simulink model "SolarPowerComp"  (R2024b)
settings: Solver=VariableStepAuto  StartTime=0.0  StopTime=10  RelTol=1e-3
undefined symbols (not defined in the file): Acid, Lead
libraries: spsSeriesRLCBranchLib x8, spsCurrentMeasurementLib x3, spsPWMGeneratorDCDCLib x2, spsDiodeLib x2, spsMosfetLib x2, spsVoltageMeasurementLib x2, spsBatteryLib x1, spsGroundLib x1, spsPVArrayLib x1, sps_lib x1
settings Model: Creator=joshbenner  LastModifiedBy=joshbenner
settings SolverCC: ZeroCrossAlgorithm=Adaptive
settings DebuggingCC: MaskedZcDiagnostic=none  IgnoredZcDiagnostic=none

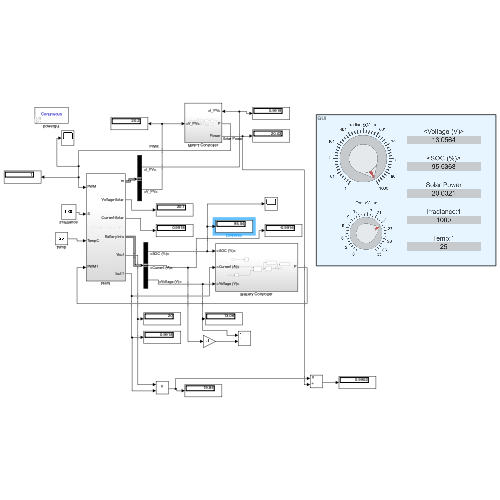
[thumbnail: Simulink's stored preview of the top-level diagram]
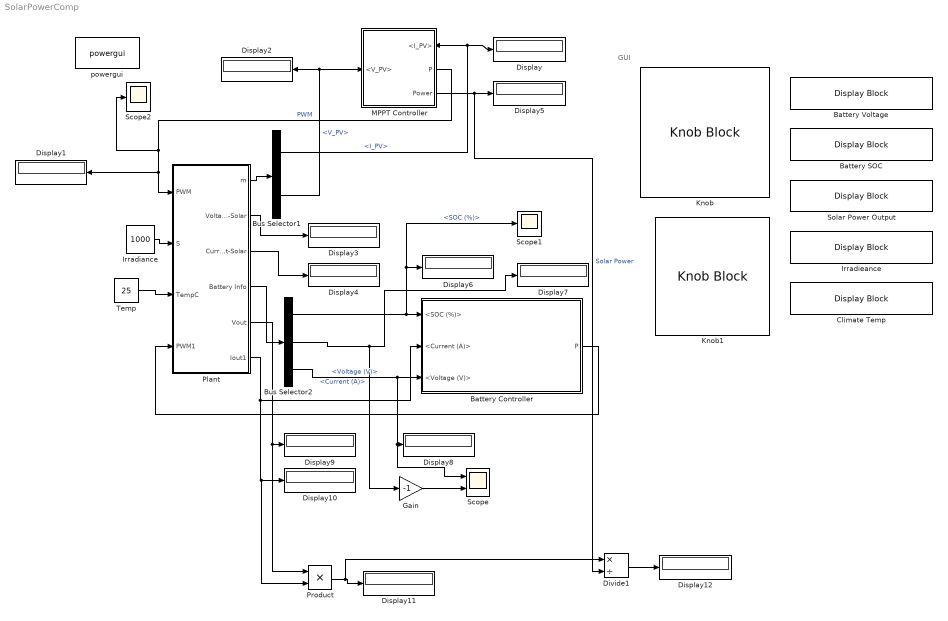
== system SolarPowerComp ==
  note: GUI
  Battery Controller : Subsystem
  Battery SOC : DisplayBlock  Transparency=1
  Battery Voltage : DisplayBlock  Transparency=1
  Bus Selector1 : BusSelector  OutputSignals=I_PV,V_PV
  Bus Selector2 : BusSelector  OutputSignals=SOC (%),Current (A),Voltage (V)
  Climate Temp : DisplayBlock  Transparency=1
  Display{,1..12} (13 alike) : Display
  Divide1 : Product  Inputs=*/
  Gain : Gain  Gain=-1
  Irradiance : Constant  Value=1000
  Irradieance : DisplayBlock  Transparency=1
  Knob : KnobBlock  ScaleMin=1  ScaleMax=1000
  Knob1 : KnobBlock  ScaleMax=35
  MPPT Controller : Subsystem
      settings: PortSchema="{\"entries\":[{\"content\":{\"sides\":[{\"content\":{\"connectorIds\":[\"In1\"]},\"type\":\"ConnectorPlacement.EquallySpacedRectSide\",\"uuid\":\"d3d26d18-f1d7-4526-bab1-51f87aba0634\"},{\"content\":{\"connectorIds\":[\"In2\",\"Out1\",\"Out2\"],\"side\":\"RIGHT\"},\"type\":\"ConnectorPlacement.EquallySpacedRectSide\",\"uuid\":\"345d964f-69df-4ff4-99f4-8db1e101ec0e\"},{\"content\":{\"side\":\"TOP\"},\"type\":\"ConnectorPlacement.EquallySpacedRectSide\",\"uuid\":\"81ceea76-a4b6-4476-a125-099e7862c238\"}]},\"type\":\"ConnectorPlacement.EquallySpacedConnector\",\"uuid\":\"a527d310-72d2-41d9-baeb-0576d2e35a0d\"}],\"packageUris\":[\"http://schema.mathworks.com/mf0/Connector/R2020b\"],\"version\":\"1.0\"}"
  Plant : Subsystem
  Product : Product
  Scope : Scope  NumInputPorts=2
  Scope1 : Scope
  Scope2 : Scope
  Solar Power Output : DisplayBlock  Transparency=1
  Temp : Constant  Value=25
  powergui : sps_lib/powergui  Priority=1  SimulationMode=Continuous  SampleTime=1e-6  frequency=60  Iterations=50  frequencyindice=0  Pbase=100e6  ErrMax=1e-4  UnitsV=kV  UnitsW=MW  buscounter=0  FunctionMessages=off  echomessages=off  EnableUseOfTLC=off  CurrentSourceSwitches=off  DisableSnubberDevices=off  DisableRonSwitches=off  DisableVfSwitches=off  DisplayEquations=off  AutomaticDiscreteSolvers=off  SolverType=Tustin/Backward Euler (TBE)  Interpol=off  ExternalGateDelay=off  methode=off  Ts=100  x0status=blocks  SPID=on  SwTol=0  HookPort=off  NonlinearTolerance=1e-4  nMaxIteration=100  ContinueOnMaxIteration=off  RestoreLinks=warning  ResistiveCurrentMeasurement=off  Frange=[0:2:500]  Ylog=off  Xlog=on  ShowGrid=off  save=off  variable=ZData  structure=0  ZoomFFT=off  StartTime=0.0  cycles=1  DisplayStyle=1  fundamental=60  FreqAxis=off  MaxFrequency=1000  frequencyindicesteady=1  RmsSteady=1  display=off
  wires:
  Bus Selector1/2 -> MPPT Controller/1(<V_PV>), Display2/1  "<V_PV>"
  Bus Selector1/1 -> MPPT Controller/2(<I_PV>), Display/1  "<I_PV>"
  MPPT Controller/1(P) -> Scope2/1, Display1/1, Plant/1(PWM)  "PWM"
  Temp/1 -> Plant/3(TempC)
  Plant/1(m) -> Bus Selector1/1
  Irradiance/1 -> Plant/2(S)
  MPPT Controller/2(Power) -> Divide1/2, Display5/1  "Solar Power"
  Plant/2(Voltage-Solar) -> Display3/1
  Plant/3(Current-Solar) -> Display4/1
  Plant/4(Battery Info) -> Bus Selector2/1
  Bus Selector2/1 -> Battery Controller/1(<SOC (%)>), Scope1/1, Display6/1  "<SOC (%)>"
  Bus Selector2/2 -> Gain/1, Display7/1  "<Current (A)>"
  Bus Selector2/3 -> Battery Controller/3(<Voltage (V)>), Scope/1, Display8/1  "<Voltage (V)>"
  Battery Controller/1(P) -> Plant/4(PWM1)
  Plant/5(Vout) -> Product/1, Display9/1
  Plant/6(Iout1) -> Battery Controller/2(<Current (A)>), Product/2, Display10/1
  Gain/1 -> Scope/2
  Product/1 -> Divide1/1, Display11/1
  Divide1/1 -> Display12/1

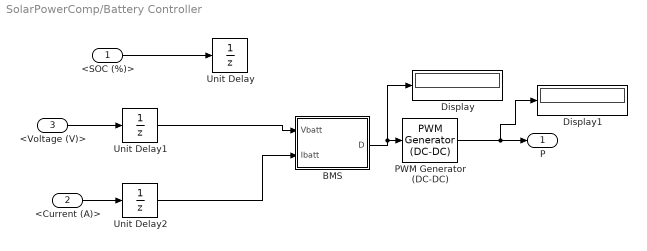
== system SolarPowerComp/Battery Controller ==
  <SOC (%)> : Inport
  <Current (A)> : Inport  Port=2
  <Voltage (V)> : Inport  Port=3
  BMS : MATLAB Function  TreatAsAtomicUnit=on
  Display : Display
  Display1 : Display
  PWM Generator (DC-DC) : spsPWMGeneratorDCDCLib/PWM Generator (DC-DC)  Fsw=100000  Ts=.000005
  Unit Delay : UnitDelay  SampleTime=-1  HasFrameUpgradeWarning=on
  Unit Delay1 : UnitDelay  SampleTime=-1  HasFrameUpgradeWarning=on
  Unit Delay2 : UnitDelay  SampleTime=-1  HasFrameUpgradeWarning=on
  P : Outport
  wires:
  PWM Generator (DC-DC)/1 -> Display1/1, P/1
  BMS/1(D) -> Display/1, PWM Generator (DC-DC)/1
  <SOC (%)>/1 -> Unit Delay/1
  <Voltage (V)>/1 -> Unit Delay1/1
  <Current (A)>/1 -> Unit Delay2/1
  Unit Delay1/1 -> BMS/1(Vbatt)
  Unit Delay2/1 -> BMS/2(Ibatt)

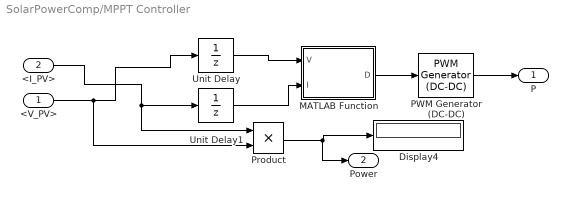
== system SolarPowerComp/MPPT Controller ==
  <V_PV> : Inport
  <I_PV> : Inport  Port=2
  Display4 : Display
  MATLAB Function : MATLAB Function  TreatAsAtomicUnit=on
  PWM Generator (DC-DC) : spsPWMGeneratorDCDCLib/PWM Generator (DC-DC)  Fsw=100000  Ts=.000005
  Product : Product
  Unit Delay : UnitDelay  SampleTime=-1  HasFrameUpgradeWarning=on
  Unit Delay1 : UnitDelay  SampleTime=-1  HasFrameUpgradeWarning=on
  P : Outport
  Power : Outport  Port=2
  wires:
  <V_PV>/1 -> Product/2, Unit Delay/1
  PWM Generator (DC-DC)/1 -> P/1
  <I_PV>/1 -> Product/1, Unit Delay1/1
  Unit Delay/1 -> MATLAB Function/1(V)
  MATLAB Function/1(D) -> PWM Generator (DC-DC)/1
  Product/1 -> Power/1, Display4/1
  Unit Delay1/1 -> MATLAB Function/2(I)

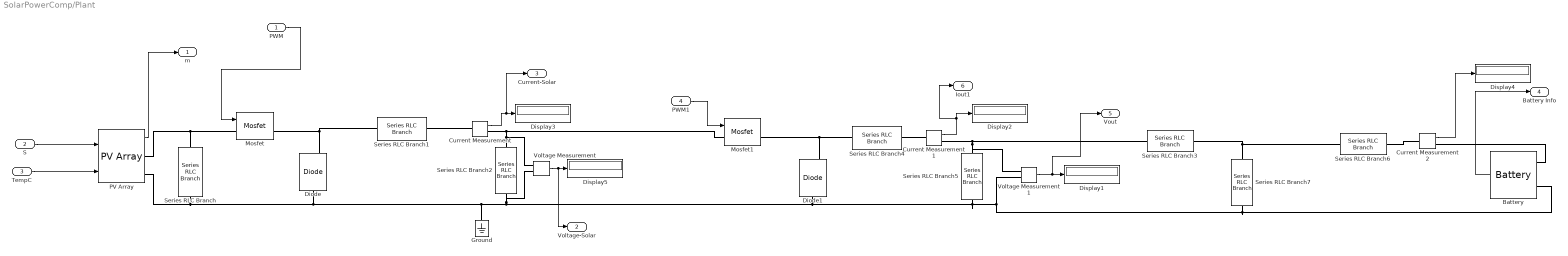
== system SolarPowerComp/Plant ==
  PWM : Inport
  S : Inport  Port=2
  TempC : Inport  Port=3
  PWM1 : Inport  Port=4
  Battery : spsBatteryLib/Battery  BatType=Lead-Acid  NomV=12  NomQ=5  SOC=95  Batt_Tr=1e-3  PresetModel=on  MaxQ=5.2083  MinV=9  FullV=13.0658  Dis_rate=1  R=0.024  Normal_OP=1.5514  expZone="[12.2171    0.0166667]"
  Current Measurement : spsCurrentMeasurementLib/Current Measurement  PhasorSimulation=off  OutputType=Complex  PSBequivalent=0
  Current Measurement1 : spsCurrentMeasurementLib/Current Measurement  PhasorSimulation=off  OutputType=Complex  PSBequivalent=0
  Current Measurement2 : spsCurrentMeasurementLib/Current Measurement  PhasorSimulation=off  OutputType=Complex  PSBequivalent=0
  Diode : spsDiodeLib/Diode  Ron=0.001  Lon=0  Vf=0.8  IC=0  UseSnubber=0  Rs=500  Cs=250e-9  Measurements=on
  Diode1 : spsDiodeLib/Diode  Ron=0.001  Lon=0  Vf=0.8  IC=0  UseSnubber=0  Rs=500  Cs=250e-9  Measurements=on
  Display{1..5} (5 alike) : Display
  Ground : spsGroundLib/Ground  LConnTagsString=a
  Mosfet : spsMosfetLib/Mosfet  Ron=0.1  Lon=0  Rd=0.01  Vfd=0  IC=0  Rs=1e5  Cs=inf  Measurements=on
  Mosfet1 : spsMosfetLib/Mosfet  Ron=0.1  Lon=0  Rd=0.01  Vfd=0  IC=0  Rs=1e5  Cs=inf  Measurements=on
  PV Array : spsPVArrayLib/PV Array  Npar=1  Nser=1  PlotType=one module @ 25 deg.C & specified irradiances  S_vec="[ 1000  500  100 ]"  Temp_C_vec="[ 45 25  ]"  ModuleName=User-defined  PlotWhenSelected=off  Pm=25.2  Ncell=60  Voc=22.41  Isc=1.54  Vm=18  Im=1.4  beta_Voc_pc=-0.36099  alpha_Isc_pc=0.102  beta_Voc=-0.080898  alpha_Isc=0.0015708  IL=1.5698  I0=5.9204e-11  nI=0.60755  Rsh=206.1422  Rs=1.1696  RobustModel=off  RobustCellTemperature=313.3991  BAL=on  Tc=1e-6  Tfilter=5e-5
  Series RLC Branch : spsSeriesRLCBranchLib/Series RLC Branch  LConnTagsString=__new0  RConnTagsString=__new0  BranchType=C  Resistance=.0001  Inductance=1e-3  SetiL0=off  InitialCurrent=0  Capacitance=1000e-6  Setx0=off  InitialVoltage=0  Measurements=None
  Series RLC Branch1 : spsSeriesRLCBranchLib/Series RLC Branch  LConnTagsString=__new0  RConnTagsString=__new0  BranchType=L  Resistance=.0001  Inductance=1e-3  SetiL0=off  InitialCurrent=0  Capacitance=1000e-6  Setx0=off  InitialVoltage=0  Measurements=None
  Series RLC Branch2 : spsSeriesRLCBranchLib/Series RLC Branch  LConnTagsString=__new0  RConnTagsString=__new0  BranchType=C  Resistance=.0001  Inductance=1e-3  SetiL0=off  InitialCurrent=0  Capacitance=20e-6  Setx0=off  InitialVoltage=0  Measurements=None
  Series RLC Branch3 : spsSeriesRLCBranchLib/Series RLC Branch  LConnTagsString=__new0  RConnTagsString=__new0  BranchType=R  Resistance=7  Inductance=1e-3  SetiL0=off  InitialCurrent=0  Capacitance=20e-6  Setx0=off  InitialVoltage=0  Measurements=None
  Series RLC Branch4 : spsSeriesRLCBranchLib/Series RLC Branch  LConnTagsString=__new0  RConnTagsString=__new0  BranchType=L  Resistance=.0001  Inductance=1e-3  SetiL0=off  InitialCurrent=0  Capacitance=1000e-6  Setx0=off  InitialVoltage=0  Measurements=None
  Series RLC Branch5 : spsSeriesRLCBranchLib/Series RLC Branch  LConnTagsString=__new0  RConnTagsString=__new0  BranchType=C  Resistance=.0001  Inductance=1e-3  SetiL0=off  InitialCurrent=0  Capacitance=20e-3  Setx0=off  InitialVoltage=0  Measurements=None
  Series RLC Branch6 : spsSeriesRLCBranchLib/Series RLC Branch  LConnTagsString=__new0  RConnTagsString=__new0  BranchType=R  Resistance=.0001  Inductance=1e-3  SetiL0=off  InitialCurrent=0  Capacitance=20e-6  Setx0=off  InitialVoltage=0  Measurements=None
  Series RLC Branch7 : spsSeriesRLCBranchLib/Series RLC Branch  LConnTagsString=__new0  RConnTagsString=__new0  BranchType=C  Resistance=.0001  Inductance=1e-3  SetiL0=off  InitialCurrent=0  Capacitance=4500e-6  Setx0=off  InitialVoltage=0  Measurements=None
  Voltage Measurement : spsVoltageMeasurementLib/Voltage Measurement  PhasorSimulation=off  OutputType=Complex  PSBequivalent=0
  Voltage Measurement1 : spsVoltageMeasurementLib/Voltage Measurement  PhasorSimulation=off  OutputType=Complex  PSBequivalent=0
  m : Outport
  Voltage-Solar : Outport  Port=2
  Current-Solar : Outport  Port=3
  Battery Info : Outport  Port=4
  Vout : Outport  Port=5
  Iout1 : Outport  Port=6
  wires:
  S/1 -> PV Array/1
  PV Array/1 -> m/1
  Voltage Measurement/1 -> Voltage-Solar/1, Display5/1
  TempC/1 -> PV Array/2
  PWM/1 -> Mosfet/1
  Current Measurement/1 -> Current-Solar/1, Display3/1
  PWM1/1 -> Mosfet1/1
  Voltage Measurement1/1 -> Vout/1, Display1/1
  Battery/1 -> Battery Info/1
  Current Measurement2/1 -> Display4/1
  Current Measurement1/1 -> Iout1/1, Display2/1
  connections:
  PV Array/RConn1 -- Series RLC Branch/LConn1 -- Mosfet/LConn1
  Diode/RConn1 -- Series RLC Branch1/LConn1 -- Mosfet/RConn1
  Series RLC Branch/RConn1 -- Ground/LConn1 -- Series RLC Branch7/RConn1 -- Battery/LConn2 -- Voltage Measurement1/LConn2 -- Series RLC Branch5/RConn1 -- Diode1/LConn1 -- Voltage Measurement/LConn2 -- Series RLC Branch2/RConn1 -- Diode/LConn1 -- PV Array/RConn2
  Series RLC Branch1/RConn1 -- Current Measurement/LConn1
  Mosfet1/RConn1 -- Diode1/RConn1 -- Series RLC Branch4/LConn1
  Series RLC Branch5/LConn1 -- Current Measurement1/RConn1 -- Series RLC Branch3/LConn1 -- Voltage Measurement1/LConn1
  Current Measurement1/LConn1 -- Series RLC Branch4/RConn1
  Current Measurement/RConn1 -- Mosfet1/LConn1 -- Voltage Measurement/LConn1 -- Series RLC Branch2/LConn1
  Current Measurement2/LConn1 -- Series RLC Branch6/RConn1
  Current Measurement2/RConn1 -- Battery/LConn1
  Series RLC Branch7/LConn1 -- Series RLC Branch3/RConn1 -- Series RLC Branch6/LConn1

== matlab function SolarPowerComp/Battery Controller/BMS ==
  settings: updateMethod=DISCRETE
  data: Vbatt input; D output; Ibatt input
function D = fcn(Vbatt, Ibatt)
% UC3906 behavioral model (PWM duty cycle control)
% Inputs:
%   Vbatt - Battery voltage
%   Ibatt - Battery current (positive = charging)
% Output:
%   D - PWM duty cycle (0–1)

% --- Parameters ---
V_bulk      = 14.5;   % Overcharge (absorption) voltage
V_float     = 13.5;   % Float voltage
V_recharge  = 12.8;   % Restart charging if voltage drops below this
I_max       = 1.9;    % Max charging current (bulk)
I_float     = 0.8;    % Float current threshold
DeltaD      = 0.001;  % Duty cycle adjustment rate
% Mode: 1=Bulk, 2=Absorption, 3=Float
persistent Duty Mode
if isempty(Duty)
    Duty = 0.5;
    Mode = 1;  % start in bulk
end

switch Mode
    case 1  % Bulk
        if (Vbatt >= V_bulk)
            Mode = 2; % Absorption
        end
    case 2  % Absorption
        if (Ibatt <= I_float)
            Mode = 3; % Float
        end
    case 3  % Float
        if (Vbatt <= V_recharge)
            Mode = 1; % Bulk
        end
end

% --- Control Logic per Mode ---
switch Mode
    case 1  % Bulk: constant current
        if (Ibatt < I_max)
            Duty = Duty + DeltaD;
        else
            Duty = Duty - DeltaD;
        end
    case 2  % Absorption: constant voltage
        if (Vbatt < V_bulk)
            Duty = Duty + DeltaD;
        else
            Duty = Duty - DeltaD;
        end
    case 3  % Float: maintain float voltage
        if (Vbatt < V_float)
            Duty = Duty + DeltaD;
        else
            Duty = Duty - DeltaD;
        end
end

Duty = max(0, min(1, Duty));
D = Duty;

== matlab function SolarPowerComp/MPPT Controller/MATLAB Function ==
  settings: updateMethod=DISCRETE
  data: V input; D output; I input
function D = fcn(V, I)
persistent Duty Vold Iold
deltaD = 0.001;

% Initialize persistent variables
if isempty(Duty)
    Duty = 0.5;
    Vold = V;
    Iold = I;
end

Pnew = V * I;
Pold = Vold * Iold;

% Compute deltas
dP = Pnew - Pold;
dV = V - Vold;

% Perturb and observe logic
if dP > 0
    % Power increased
    if dV > 0
        Duty = Duty - deltaD; % move same direction
    else
        Duty = Duty + deltaD; % reverse direction
    end
elseif dP < 0
    % Power decreased
    if dV > 0
        Duty = Duty +deltaD;
    else
        Duty = Duty - deltaD;
    end
else
    % No change in power — keep duty same
    Duty = Duty;
end

% Limit duty between 0 and 1
Duty = max(0, min(1, Duty));

% Update old values
Vold = V;
Iold = I;

% Return updated duty
D = Duty;
end
